simulink model "DiscreteDiscreteEj2"  (R2017b)
settings: Solver=VariableStepAuto  StartTime=0.0  StopTime=10.0  RelTol=1e-3
values from neighbouring files (symbols this model uses):
  ki = double(ki)    [DiscreteDiscreteEj2Matlab.m]    (also in DiscreteDiscreteMatlab.m; P_I_D.m = eval(S.ki))
  ki2 = double(ki2)    [DiscreteDiscreteEj2Matlab.m]    (also in P_I_D.m = eval(S.ki2))
  ki3 = double(ki3)    [DiscreteDiscreteEj2Matlab.m]
  ki4 = double(ki4)    [DiscreteDiscreteEj2Matlab.m]
  PIDZn = PIDZ.num{1}    [DiscreteDiscreteEj2Matlab.m]
  r1 = x(2)    [DiscreteDiscreteEj2Matlab.m]    (also in DiscreteDiscreteMatlab.m = x(4))
  r2 = x(3)    [DiscreteDiscreteEj2Matlab.m]    (also in DiscreteDiscreteMatlab.m = x(5))
  r3 = x(4)    [DiscreteDiscreteEj2Matlab.m]
  r4 = x(5)    [DiscreteDiscreteEj2Matlab.m]
  tm = 0.125    [DiscreteDiscreteEj2Matlab.m]    (also in DiscreteDiscreteMatlab.m = 0.25)
libraries: simulink x6
settings Model: Creator=Cx001la  LastModifiedBy=Cx001la

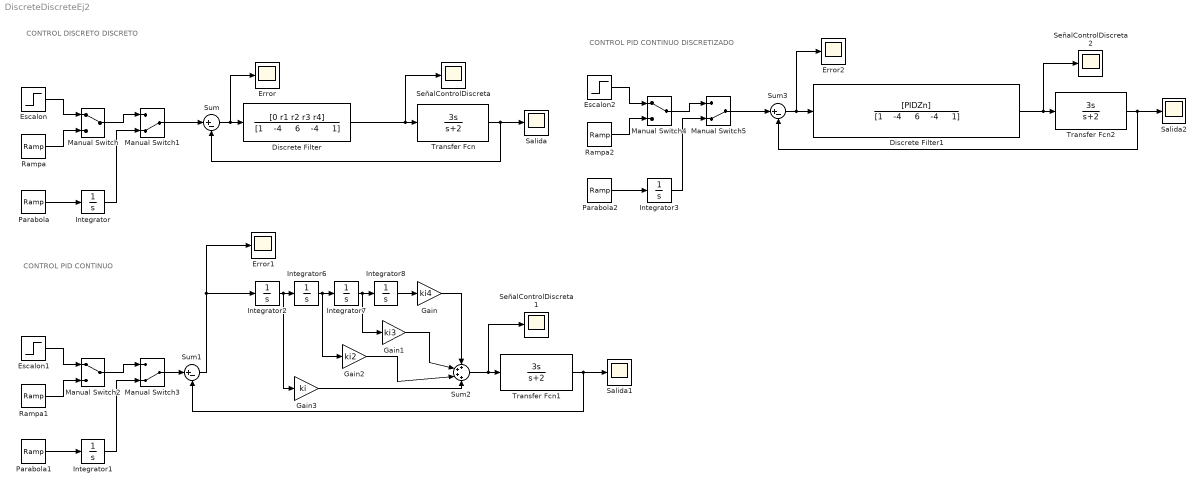
== system DiscreteDiscreteEj2 ==
  note: CONTROL DISCRETO DISCRETO
  note: CONTROL PID CONTINUO
  note: CONTROL PID CONTINUO DISCRETIZADO
  Discrete Filter : DiscreteFilter  Numerator=[0 r1 r2 r3 r4]  Denominator="[1    -4     6    -4     1]"  SampleTime=tm
  Discrete Filter1 : DiscreteFilter  Numerator=[PIDZn]  Denominator="[1    -4     6    -4     1]"  SampleTime=tm
  Error : Scope
  Error1 : Scope
  Error2 : Scope
  Escalon : Step  SampleTime=0
  Escalon1 : Step  SampleTime=0
  Escalon2 : Step  SampleTime=0
  Gain : Gain  Gain=ki4
  Gain1 : Gain  Gain=ki3
  Gain2 : Gain  Gain=ki2
  Gain3 : Gain  Gain=ki
  Integrator{,1..3,6..8} (7 alike) : Integrator
  Manual Switch : ManualSwitch
  Manual Switch1 : ManualSwitch  CurrentSetting=0
  Manual Switch2 : ManualSwitch
  Manual Switch3 : ManualSwitch  CurrentSetting=0
  Manual Switch4 : ManualSwitch
  Manual Switch5 : ManualSwitch  CurrentSetting=0
  Parabola : simulink/Sources/Ramp  slope=1  start=0  X0=0
  Parabola1 : simulink/Sources/Ramp  slope=1  start=0  X0=0
  Parabola2 : simulink/Sources/Ramp  slope=1  start=0  X0=0
  Rampa : simulink/Sources/Ramp  slope=1  start=0  X0=0
  Rampa1 : simulink/Sources/Ramp  slope=1  start=0  X0=0
  Rampa2 : simulink/Sources/Ramp  slope=1  start=0  X0=0
  Salida : Scope
  Salida1 : Scope
  Salida2 : Scope
  SeñalControlDiscreta : Scope
  SeñalControlDiscreta1 : Scope
  SeñalControlDiscreta2 : Scope
  Sum : Sum  Inputs=|+-
  Sum1 : Sum  Inputs=|+-
  Sum2 : Sum  Inputs=++++
  Sum3 : Sum  Inputs=|+-
  Transfer Fcn : TransferFcn  Numerator=[3 0]  Denominator=[1 2 ]
  Transfer Fcn1 : TransferFcn  Numerator=[3 0]  Denominator=[1 2 ]
  Transfer Fcn2 : TransferFcn  Numerator=[3 0]  Denominator=[1 2 ]
  wires:
  Discrete Filter/1 -> SeñalControlDiscreta/1, Transfer Fcn/1
  Escalon/1 -> Manual Switch/1
  Transfer Fcn/1 -> Salida/1, Sum/2
  Rampa/1 -> Manual Switch/2
  Sum/1 -> Error/1, Discrete Filter/1
  Parabola/1 -> Integrator/1
  Manual Switch/1 -> Manual Switch1/1
  Manual Switch1/1 -> Sum/1
  Integrator/1 -> Manual Switch1/2
  Parabola1/1 -> Integrator1/1
  Manual Switch3/1 -> Sum1/1
  Sum2/1 -> SeñalControlDiscreta1/1, Transfer Fcn1/1
  Rampa1/1 -> Manual Switch2/2
  Escalon1/1 -> Manual Switch2/1
  Manual Switch2/1 -> Manual Switch3/1
  Integrator1/1 -> Manual Switch3/2
  Transfer Fcn1/1 -> Salida1/1, Sum1/2
  Integrator8/1 -> Gain/1
  Sum1/1 -> Integrator2/1, Error1/1
  Integrator2/1 -> Gain3/1, Integrator6/1
  Integrator6/1 -> Gain2/1, Integrator7/1
  Integrator7/1 -> Gain1/1, Integrator8/1
  Gain/1 -> Sum2/1
  Gain1/1 -> Sum2/2
  Gain2/1 -> Sum2/3
  Gain3/1 -> Sum2/4
  Parabola2/1 -> Integrator3/1
  Manual Switch5/1 -> Sum3/1
  Discrete Filter1/1 -> SeñalControlDiscreta2/1, Transfer Fcn2/1
  Rampa2/1 -> Manual Switch4/2
  Sum3/1 -> Error2/1, Discrete Filter1/1
  Escalon2/1 -> Manual Switch4/1
  Manual Switch4/1 -> Manual Switch5/1
  Integrator3/1 -> Manual Switch5/2
  Transfer Fcn2/1 -> Salida2/1, Sum3/2
